simulink model "ROBOT"  (R2017a)
settings: Solver=VariableStepAuto  StartTime=0.0  StopTime=inf  MaxStep=0.05  RelTol=1e-3
model workspace: external: MATLAB File C:\Users\Robotic\Desktop\robot_solid\robot matlab\新建文件夹\ROBOT_DataFile.m (data not in the file)
values from neighbouring files (symbols this model uses):
  m = linspace(SD_4(1,30),SD_4(1,2),10)    [Gait_walking_go.m]
  X = A\B    [orbit_function.m]
  Y = 25*sin(2*pi/T*t)    [Gait_walkin.m]    (also in Gait_walking.m = 5*sin(2*pi/T*t); Gait_walking_go.m = 40*sin(2*pi/T*t))
undefined symbols (not defined in the file or in its folder): smiData, Z
libraries: sm_lib x579, nesl_utility x24, sldrtlib x1
(part 1 of 11)
settings Model: Creator=Robotic  LastModifiedBy=Administrator

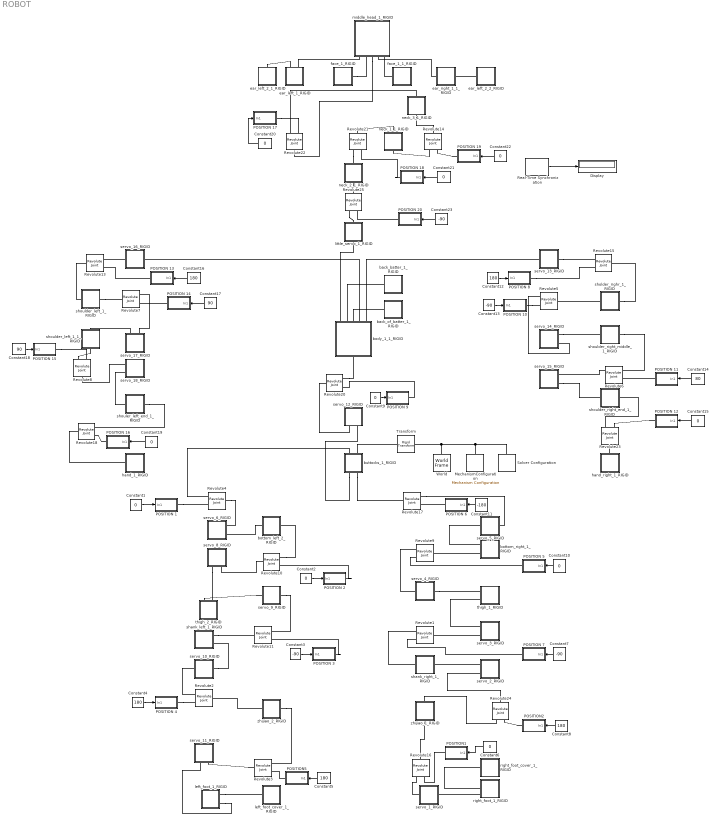
== system ROBOT ==
  Constant{1..2,6,9..10,15,19..22} (10 alike) : Constant  Value=0
  Constant11 : Constant  Value=-180
  Constant{4..5,8,12,16} (5 alike) : Constant  Value=180
  Constant{3,7,13,23} (4 alike) : Constant  Value=-90
  Constant14 : Constant  Value=80
  Constant17 : Constant  Value=90
  Constant18 : Constant  Value=90
  Display : Display
  MechanismConfiguration : sm_lib/Utilities/Mechanism Configuration  UniformGravity=Constant  GravityVector=[0 -9.80665 0]  GravityUnits=m/s^2  LinearizationDelta=0.001
  POSITION 1 : Subsystem
  POSITION 10 : Subsystem
  POSITION 11 : Subsystem
  POSITION 12 : Subsystem
  POSITION 13 : Subsystem
  POSITION 14 : Subsystem
  POSITION 15 : Subsystem
  POSITION 16 : Subsystem
  POSITION 17 : Subsystem
  POSITION 18 : Subsystem
  POSITION 19 : Subsystem
  POSITION 2 : Subsystem
  POSITION 20 : Subsystem
  POSITION 3 : Subsystem
  POSITION 4 : Subsystem
  POSITION 5 : Subsystem
  POSITION 6 : Subsystem
  POSITION 7 : Subsystem
  POSITION 8 : Subsystem
  POSITION 9 : Subsystem
  POSITION1 : Subsystem
  POSITION2 : Subsystem
  POSITION5 : Subsystem
  Real-Time Synchronization : sldrtlib/Real-Time Synchronization  SampleTime=0.1  MaxMissedTicks=100  ShowMissedTicks=on  YieldWhenWaiting=off
  Revolute{1..3,5,7..9,11,13..18,21..25} (19 alike) : sm_lib/Joints/Revolute Joint  SenseConstraintForce=off  SenseConstraintForceX=off  SenseConstraintForceY=off  SenseConstraintForceZ=off  SenseConstraintTorque=off  SenseConstraintTorqueX=off  SenseConstraintTorqueY=off  SenseConstraintTorqueZ=off  SenseTotalForce=off  SenseTotalForceX=off  SenseTotalForceY=off  SenseTotalForceZ=off  SenseTotalTorque=off  SenseTotalTorqueX=off  SenseTotalTorqueY=off  SenseTotalTorqueZ=off  CompositeWrenchDir=FollowerOnBase  CompositeWrenchFrame=BaseFrame  EquilibriumPosition=0  EquilibriumPositionUnits=rad  SpringStiffness=0  SpringStiffnessUnits=N*m/rad  DampingCoefficient=0  DampingCoefficientUnits=N*m/(rad/s)  TorqueActuationMode=ComputedTorque  MotionActuationMode=InputMotion  SensePosition=off  SenseVelocity=off  SenseAcceleration=off  SenseTorqueForce=off  PositionTargetSpecify=off  PositionTargetPriority=Low  PositionTargetValue=smiData.RevoluteJoint(2).Rz.Pos  PositionTargetValueUnits=deg  VelocityTargetSpecify=off  VelocityTargetPriority=High  VelocityTargetValue=0  VelocityTargetValueUnits=deg/s
  Revolute10 : sm_lib/Joints/Revolute Joint  SenseConstraintForce=off  SenseConstraintForceX=off  SenseConstraintForceY=off  SenseConstraintForceZ=off  SenseConstraintTorque=off  SenseConstraintTorqueX=off  SenseConstraintTorqueY=off  SenseConstraintTorqueZ=off  SenseTotalForce=off  SenseTotalForceX=off  SenseTotalForceY=off  SenseTotalForceZ=off  SenseTotalTorque=off  SenseTotalTorqueX=off  SenseTotalTorqueY=off  SenseTotalTorqueZ=off  CompositeWrenchDir=FollowerOnBase  CompositeWrenchFrame=BaseFrame  EquilibriumPosition=0  EquilibriumPositionUnits=rad  SpringStiffness=0  SpringStiffnessUnits=N*m/rad  DampingCoefficient=0  DampingCoefficientUnits=N*m/(rad/s)  TorqueActuationMode=ComputedTorque  MotionActuationMode=InputMotion  SensePosition=off  SenseVelocity=off  SenseAcceleration=off  SenseTorqueForce=off  PositionTargetSpecify=on  PositionTargetPriority=Low  PositionTargetValue=smiData.RevoluteJoint(2).Rz.Pos  PositionTargetValueUnits=deg  VelocityTargetSpecify=off  VelocityTargetPriority=High  VelocityTargetValue=0  VelocityTargetValueUnits=deg/s
  Revolute20 : sm_lib/Joints/Revolute Joint  SenseConstraintForce=off  SenseConstraintForceX=off  SenseConstraintForceY=off  SenseConstraintForceZ=off  SenseConstraintTorque=off  SenseConstraintTorqueX=off  SenseConstraintTorqueY=off  SenseConstraintTorqueZ=off  SenseTotalForce=off  SenseTotalForceX=off  SenseTotalForceY=off  SenseTotalForceZ=off  SenseTotalTorque=off  SenseTotalTorqueX=off  SenseTotalTorqueY=off  SenseTotalTorqueZ=off  CompositeWrenchDir=FollowerOnBase  CompositeWrenchFrame=BaseFrame  EquilibriumPosition=0  EquilibriumPositionUnits=rad  SpringStiffness=0  SpringStiffnessUnits=N*m/rad  DampingCoefficient=0  DampingCoefficientUnits=N*m/(rad/s)  TorqueActuationMode=ComputedTorque  MotionActuationMode=InputMotion  SensePosition=off  SenseVelocity=off  SenseAcceleration=off  SenseTorqueForce=off  PositionTargetSpecify=on  PositionTargetPriority=Low  PositionTargetValue=smiData.RevoluteJoint(2).Rz.Pos  PositionTargetValueUnits=deg  VelocityTargetSpecify=off  VelocityTargetPriority=High  VelocityTargetValue=0  VelocityTargetValueUnits=deg/s
  Revolute4 : sm_lib/Joints/Revolute Joint  SenseConstraintForce=off  SenseConstraintForceX=off  SenseConstraintForceY=off  SenseConstraintForceZ=off  SenseConstraintTorque=off  SenseConstraintTorqueX=off  SenseConstraintTorqueY=off  SenseConstraintTorqueZ=off  SenseTotalForce=off  SenseTotalForceX=off  SenseTotalForceY=off  SenseTotalForceZ=off  SenseTotalTorque=off  SenseTotalTorqueX=off  SenseTotalTorqueY=off  SenseTotalTorqueZ=off  CompositeWrenchDir=FollowerOnBase  CompositeWrenchFrame=BaseFrame  EquilibriumPosition=0  EquilibriumPositionUnits=rad  SpringStiffness=0  SpringStiffnessUnits=N*m/rad  DampingCoefficient=0  DampingCoefficientUnits=N*m/(rad/s)  TorqueActuationMode=ComputedTorque  MotionActuationMode=InputMotion  SensePosition=off  SenseVelocity=off  SenseAcceleration=off  SenseTorqueForce=off  PositionTargetSpecify=on  PositionTargetPriority=Low  PositionTargetValue=smiData.RevoluteJoint(2).Rz.Pos  PositionTargetValueUnits=deg  VelocityTargetSpecify=off  VelocityTargetPriority=High  VelocityTargetValue=0  VelocityTargetValueUnits=deg/s
  Revolute6 : sm_lib/Joints/Revolute Joint  SenseConstraintForce=off  SenseConstraintForceX=off  SenseConstraintForceY=off  SenseConstraintForceZ=off  SenseConstraintTorque=off  SenseConstraintTorqueX=off  SenseConstraintTorqueY=off  SenseConstraintTorqueZ=off  SenseTotalForce=off  SenseTotalForceX=off  SenseTotalForceY=off  SenseTotalForceZ=off  SenseTotalTorque=off  SenseTotalTorqueX=off  SenseTotalTorqueY=off  SenseTotalTorqueZ=off  CompositeWrenchDir=FollowerOnBase  CompositeWrenchFrame=BaseFrame  EquilibriumPosition=0  EquilibriumPositionUnits=rad  SpringStiffness=0  SpringStiffnessUnits=N*m/rad  DampingCoefficient=0  DampingCoefficientUnits=N*m/(rad/s)  TorqueActuationMode=ComputedTorque  MotionActuationMode=InputMotion  SensePosition=on  SenseVelocity=off  SenseAcceleration=off  SenseTorqueForce=off  PositionTargetSpecify=off  PositionTargetPriority=Low  PositionTargetValue=smiData.RevoluteJoint(2).Rz.Pos  PositionTargetValueUnits=deg  VelocityTargetSpecify=off  VelocityTargetPriority=High  VelocityTargetValue=0  VelocityTargetValueUnits=deg/s
  Solver Configuration : nesl_utility/Solver Configuration  PhysicalDomain=network_engine_domain  SubClassName=solver  LeftPortType=input  RightPortType=generic  Accelerate=off  Tones=[]  Harmonics=[]  SimulateNoise=off  Profile=off  UseLocalSampling=off  EnableSwitchedLinearOptims=on  FrequencyDomain=off  UseCCode=off  RelTol=0.001  AbsTol=1e-06  MinStep=1e-09  ToWorkspace=off  RevertToSquareIcSolve=off  NumHomotopyIterations=100  PhasorMode=off  PhasorModeNumHarmonics=1  OverrideAbsTol=off  DoDC=off  ResidualTolerance=1e-09  UseLocalSolver=off  LocalSolverChoice=NE_BACKWARD_EULER_ADVANCER  LocalSolverSampleTime=0.001  DoFixedCost=off  MaxNonlinIter=3  MaxModeIter=2  LinearAlgebra=Sparse  DelaysMemoryBudget=1024  AutomaticFiltering=on  FilteringTimeConstant=0.001
  Transform : sm_lib/Frames and Transforms/Rigid Transform  TranslationMethod=Cartesian  TranslationStandardOffset=0  TranslationLengthUnit=mm  TranslationStandardAxis=+Z  TranslationCartesianOffset=smiData.RigidTransform(235).translation  TranslationROffset=0  TranslationROffsetUnits=m  TranslationZOffset=0  TranslationZOffsetUnits=m  TranslationThetaOffset=0  TranslationThetaOffsetUnits=deg  RotationMethod=ArbitraryAxis  RotationAngleUnits=rad  RotationStandardAxis=+Z  RotationAngle=smiData.RigidTransform(235).angle  RotationArbitraryAxis=smiData.RigidTransform(235).axis  FollAlignAxisA=+X  BaseAlignAxisA=+Y  FollAlignAxisB=+Y  BaseAlignAxisB=+Z  RotationSequenceAxes=FollowerAxes  RotationSequence=XYX  RotationSequenceAngles=[0 0 0]  RotationSequenceAnglesUnits=deg  RotationMatrix=[1 0 0; 0 1 0; 0 0 1]
  World : sm_lib/Frames and Transforms/World Frame
  back_batter_1_RIGID : Subsystem
  back_of_batter_1_RIGID : Subsystem
  body_1_1_RIGID : Subsystem
  bottom_left_2_RIGID : Subsystem
  bottom_right_1_RIGID : Subsystem
  buttocks_1_RIGID : Subsystem
  ear_left_1_RIGID : Subsystem
  ear_left_2_1_RIGID : Subsystem
  ear_left_2_2_RIGID : Subsystem
  ear_right_1_1_RIGID : Subsystem
  face_1_1_RIGID : Subsystem
  face_1_RIGID : Subsystem
  hand_1_RIGID : Subsystem
  hand_right_1_RIGID : Subsystem
  left_foot_1_RIGID : Subsystem
  left_foot_cover_1_RIGID : Subsystem
  little_servo_1_RIGID : Subsystem
  middle_head_1_RIGID : Subsystem
  neck_1_1_RIGID : Subsystem
  neck_2_1_RIGID : Subsystem
  neck_3_1_RIGID : Subsystem
  right_foot_1_RIGID : Subsystem
  right_foot_cover_1_RIGID : Subsystem
  servo_10_RIGID : Subsystem
  servo_11_RIGID : Subsystem
  servo_12_RIGID : Subsystem
  servo_13_RIGID : Subsystem
  servo_14_RIGID : Subsystem
  servo_15_RIGID : Subsystem
  servo_16_RIGID : Subsystem
  servo_17_RIGID : Subsystem
  servo_18_RIGID : Subsystem
  servo_1_RIGID : Subsystem
  servo_2_RIGID : Subsystem
  servo_3_RIGID : Subsystem
  servo_4_RIGID : Subsystem
  servo_5_RIGID : Subsystem
  servo_6_RIGID : Subsystem
  servo_8_RIGID : Subsystem
  servo_9_RIGID : Subsystem
  shank_left_1_RIGID : Subsystem
  shank_right_1_RIGID : Subsystem
  sholder_righr_1_RIGID : Subsystem
  shoulder_left_1_1_RIGID : Subsystem
  shoulder_left_1_RIGID : Subsystem
  shoulder_right_end_1_RIGID : Subsystem
  shoulder_right_middle_1_RIGID : Subsystem
  shouler_left_end_1_RIGID : Subsystem
  thigh_1_RIGID : Subsystem
  thigh_2_RIGID : Subsystem
  zhijiao_1_RIGID : Subsystem
  zhijiao_2_RIGID : Subsystem
  wires:
  Constant7/1 -> POSITION 7/1(In1)
  Constant9/1 -> POSITION 9/1(In1)
  Constant1/1 -> POSITION 1/1(In1)
  Constant2/1 -> POSITION 2/1(In1)
  Constant3/1 -> POSITION 3/1(In1)
  Constant4/1 -> POSITION 4/1(In1)
  Constant5/1 -> POSITION5/1(In1)
  Constant6/1 -> POSITION1/1(In1)
  Constant8/1 -> POSITION2/1(In1)
  Constant10/1 -> POSITION 5/1(In1)
  Constant11/1 -> POSITION 6/1(In1)
  Constant12/1 -> POSITION 8/1(In1)
  Constant13/1 -> POSITION 10/1(In1)
  Constant14/1 -> POSITION 11/1(In1)
  Constant15/1 -> POSITION 12/1(In1)
  Constant16/1 -> POSITION 13/1(In1)
  Constant17/1 -> POSITION 14/1(In1)
  Constant18/1 -> POSITION 15/1(In1)
  Constant19/1 -> POSITION 16/1(In1)
  Constant20/1 -> POSITION 17/1(In1)
  Constant21/1 -> POSITION 18/1(In1)
  Constant22/1 -> POSITION 19/1(In1)
  Constant23/1 -> POSITION 20/1(In1)
  Real-Time Synchronization/1 -> Display/1
  connections:
  left_foot_1_RIGID/LConn2 -- servo_11_RIGID/LConn1
  body_1_1_RIGID/LConn5 -- servo_13_RIGID/LConn1
  servo_13_RIGID/RConn1 -- Revolute15/LConn1
  sholder_righr_1_RIGID/LConn1 -- Revolute15/RConn1
  sholder_righr_1_RIGID/RConn1 -- Revolute5/RConn1
  Revolute5/LConn1 -- servo_14_RIGID/LConn2
  servo_15_RIGID/LConn2 -- shoulder_right_end_1_RIGID/LConn1
  body_1_1_RIGID/LConn4 -- servo_16_RIGID/LConn1
  zhijiao_1_RIGID/LConn1 -- Revolute16/RConn1
  servo_16_RIGID/RConn1 -- Revolute13/LConn1
  shoulder_left_1_RIGID/LConn1 -- Revolute13/RConn1
  shoulder_left_1_RIGID/RConn1 -- Revolute7/RConn1
  servo_17_RIGID/LConn2 -- Revolute7/LConn1
  servo_18_RIGID/LConn2 -- shouler_left_end_1_RIGID/LConn1
  back_of_batter_1_RIGID/LConn1 -- body_1_1_RIGID/LConn3
  right_foot_1_RIGID/LConn3 -- servo_1_RIGID/LConn1
  right_foot_1_RIGID/LConn2 -- right_foot_cover_1_RIGID/LConn1
  servo_2_RIGID/LConn1 -- shank_right_1_RIGID/LConn1
  servo_3_RIGID/LConn1 -- thigh_1_RIGID/LConn2
  zhijiao_1_RIGID/RConn1 -- Revolute24/LConn1
  shank_right_1_RIGID/RConn1 -- Revolute1/LConn1
  servo_3_RIGID/LConn2 -- Revolute1/RConn1
  servo_4_RIGID/LConn1 -- thigh_1_RIGID/LConn1
  bottom_left_2_RIGID/LConn1 -- servo_6_RIGID/LConn2
  Revolute10/LConn1 -- bottom_left_2_RIGID/RConn1
  Revolute10/RConn1 -- servo_8_RIGID/LConn2
  servo_8_RIGID/LConn1 -- thigh_2_RIGID/LConn2
  servo_9_RIGID/LConn1 -- thigh_2_RIGID/LConn1
  servo_9_RIGID/RConn1 -- Revolute11/LConn1
  shank_left_1_RIGID/LConn1 -- Revolute11/RConn1
  servo_2_RIGID/LConn2 -- Revolute24/RConn1
  back_batter_1_RIGID/LConn1 -- body_1_1_RIGID/LConn2
  shouler_left_end_1_RIGID/RConn1 -- Revolute18/LConn1
  hand_1_RIGID/LConn1 -- Revolute18/RConn1
  left_foot_1_RIGID/LConn1 -- left_foot_cover_1_RIGID/LConn1
  Revolute23/LConn1 -- shoulder_right_end_1_RIGID/RConn1
  hand_right_1_RIGID/LConn1 -- Revolute23/RConn1
  body_1_1_RIGID/LConn1 -- little_servo_1_RIGID/LConn1
  Revolute25/LConn1 -- little_servo_1_RIGID/RConn1
  Revolute25/RConn1 -- neck_2_1_RIGID/LConn1
  buttocks_1_RIGID/LConn1 -- servo_12_RIGID/LConn2
  Revolute17/LConn1 -- servo_5_RIGID/RConn1
  buttocks_1_RIGID/LConn2 -- Revolute17/RConn1
  Revolute4/RConn1 -- servo_6_RIGID/LConn1
  face_1_1_RIGID/LConn1 -- middle_head_1_RIGID/LConn5
  servo_4_RIGID/RConn1 -- Revolute9/LConn1
  bottom_right_1_RIGID/LConn2 -- Revolute9/RConn1
  bottom_right_1_RIGID/LConn1 -- servo_5_RIGID/LConn1
  servo_17_RIGID/LConn1 -- shoulder_left_1_1_RIGID/LConn1
  shoulder_left_1_1_RIGID/RConn1 -- Revolute8/LConn1
  zhijiao_2_RIGID/LConn1 -- Revolute2/RConn1
  servo_18_RIGID/LConn1 -- Revolute8/RConn1
  ear_right_1_1_RIGID/LConn1 -- middle_head_1_RIGID/LConn4
  face_1_RIGID/LConn1 -- middle_head_1_RIGID/LConn2
  ear_left_1_RIGID/LConn2 -- middle_head_1_RIGID/LConn1
  neck_3_1_RIGID/RConn1 -- Revolute22/LConn1
  middle_head_1_RIGID/LConn3 -- Revolute22/RConn1
  ear_left_1_RIGID/LConn1 -- ear_left_2_1_RIGID/LConn1
  ear_left_2_2_RIGID/LConn1 -- ear_right_1_1_RIGID/RConn1
  Revolute21/LConn1 -- neck_2_1_RIGID/RConn1
  zhijiao_2_RIGID/RConn1 -- Revolute3/LConn1
  neck_1_1_RIGID/LConn1 -- Revolute21/RConn1
  Revolute14/LConn1 -- neck_1_1_RIGID/RConn1
  neck_3_1_RIGID/LConn1 -- Revolute14/RConn1
  servo_14_RIGID/LConn1 -- shoulder_right_middle_1_RIGID/LConn1
  shoulder_right_middle_1_RIGID/RConn1 -- Revolute6/LConn1
  Revolute6/RConn1 -- servo_15_RIGID/LConn1
  Revolute3/RConn1 -- servo_11_RIGID/LConn2
  servo_10_RIGID/LConn1 -- shank_left_1_RIGID/LConn2
  MechanismConfiguration/RConn1 -- Solver Configuration/RConn1 -- World/RConn1 -- Transform/LConn1
  Transform/RConn1 -- buttocks_1_RIGID/RConn2
  Revolute20/LConn1 -- body_1_1_RIGID/RConn1
  Revolute20/RConn1 -- servo_12_RIGID/LConn1
  POSITION 9/RConn1 -- Revolute20/LConn2
  buttocks_1_RIGID/RConn1 -- Revolute4/LConn1
  POSITION 1/RConn1 -- Revolute4/LConn2
  POSITION 2/RConn1 -- Revolute10/LConn2
  POSITION 3/RConn1 -- Revolute11/LConn2
  POSITION 4/RConn1 -- Revolute2/LConn2
  Revolute2/LConn1 -- servo_10_RIGID/RConn1
  POSITION5/RConn1 -- Revolute3/LConn2
  servo_1_RIGID/RConn1 -- Revolute16/LConn1
  POSITION1/RConn1 -- Revolute16/LConn2
  POSITION2/RConn1 -- Revolute24/LConn2
  POSITION 7/RConn1 -- Revolute1/LConn2
  POSITION 5/RConn1 -- Revolute9/LConn2
  POSITION 6/RConn1 -- Revolute17/LConn2
  POSITION 8/RConn1 -- Revolute15/LConn2
  POSITION 10/RConn1 -- Revolute5/LConn2
  POSITION 11/RConn1 -- Revolute6/LConn2
  POSITION 12/RConn1 -- Revolute23/LConn2
  POSITION 13/RConn1 -- Revolute13/LConn2
  POSITION 14/RConn1 -- Revolute7/LConn2
  POSITION 15/RConn1 -- Revolute8/LConn2
  POSITION 16/RConn1 -- Revolute18/LConn2
  POSITION 17/RConn1 -- Revolute22/LConn2
  POSITION 18/RConn1 -- Revolute21/LConn2
  POSITION 19/RConn1 -- Revolute14/LConn2
  POSITION 20/RConn1 -- Revolute25/LConn2

== system ROBOT/POSITION 1 ==
  In1 : Inport
  Constant : Constant  Value=0
  Gain : Gain  Gain=pi/180
  Simulink-PS Converter : nesl_utility/Simulink-PS Converter  PhysicalDomain=network_engine_domain  SubClassName=ps_input  LeftPortType=input  RightPortType=output  PseudoPeriodic=off  Frequencies=[]  NoiseDistribution=none  NoiseParameters=[]  Unit=rad  AffineConversion=off  FilteringAndDerivatives=provide  SimscapeFilterOrder=1  InputFilterTimeConstant=0.001  UdotUserProvided=0
  Subtract : Sum
  Conn1 : PMIOPort  Port=1  Side=Right
  wires:
  Gain/1 -> Simulink-PS Converter/1
  Constant/1 -> Subtract/2
  In1/1 -> Subtract/1
  Subtract/1 -> Gain/1
  connections:
  Simulink-PS Converter/RConn1 -- Conn1/RConn1

== system ROBOT/POSITION 10 ==
  In1 : Inport
  Constant : Constant  Value=0
  Gain : Gain  Gain=pi/180
  Simulink-PS Converter : nesl_utility/Simulink-PS Converter  PhysicalDomain=network_engine_domain  SubClassName=ps_input  LeftPortType=input  RightPortType=output  PseudoPeriodic=off  Frequencies=[]  NoiseDistribution=none  NoiseParameters=[]  Unit=rad  AffineConversion=off  FilteringAndDerivatives=provide  SimscapeFilterOrder=1  InputFilterTimeConstant=0.001  UdotUserProvided=0
  Subtract : Sum
  Conn1 : PMIOPort  Port=1  Side=Right
  wires:
  Gain/1 -> Simulink-PS Converter/1
  Constant/1 -> Subtract/2
  In1/1 -> Subtract/1
  Subtract/1 -> Gain/1
  connections:
  Simulink-PS Converter/RConn1 -- Conn1/RConn1

== system ROBOT/POSITION 11 ==
  In1 : Inport
  Constant : Constant  Value=0
  Gain : Gain  Gain=pi/180
  Simulink-PS Converter : nesl_utility/Simulink-PS Converter  PhysicalDomain=network_engine_domain  SubClassName=ps_input  LeftPortType=input  RightPortType=output  PseudoPeriodic=off  Frequencies=[]  NoiseDistribution=none  NoiseParameters=[]  Unit=rad  AffineConversion=off  FilteringAndDerivatives=provide  SimscapeFilterOrder=1  InputFilterTimeConstant=0.001  UdotUserProvided=0
  Subtract : Sum
  Conn1 : PMIOPort  Port=1  Side=Right
  wires:
  Gain/1 -> Simulink-PS Converter/1
  Constant/1 -> Subtract/2
  In1/1 -> Subtract/1
  Subtract/1 -> Gain/1
  connections:
  Simulink-PS Converter/RConn1 -- Conn1/RConn1

== system ROBOT/POSITION 12 ==
  In1 : Inport
  Constant : Constant  Value=0
  Gain : Gain  Gain=pi/180
  Simulink-PS Converter : nesl_utility/Simulink-PS Converter  PhysicalDomain=network_engine_domain  SubClassName=ps_input  LeftPortType=input  RightPortType=output  PseudoPeriodic=off  Frequencies=[]  NoiseDistribution=none  NoiseParameters=[]  Unit=rad  AffineConversion=off  FilteringAndDerivatives=provide  SimscapeFilterOrder=1  InputFilterTimeConstant=0.001  UdotUserProvided=0
  Subtract : Sum
  Conn1 : PMIOPort  Port=1  Side=Right
  wires:
  Gain/1 -> Simulink-PS Converter/1
  Constant/1 -> Subtract/2
  In1/1 -> Subtract/1
  Subtract/1 -> Gain/1
  connections:
  Simulink-PS Converter/RConn1 -- Conn1/RConn1

== system ROBOT/POSITION 13 ==
  In1 : Inport
  Constant : Constant  Value=0
  Gain : Gain  Gain=pi/180
  Simulink-PS Converter : nesl_utility/Simulink-PS Converter  PhysicalDomain=network_engine_domain  SubClassName=ps_input  LeftPortType=input  RightPortType=output  PseudoPeriodic=off  Frequencies=[]  NoiseDistribution=none  NoiseParameters=[]  Unit=rad  AffineConversion=off  FilteringAndDerivatives=provide  SimscapeFilterOrder=1  InputFilterTimeConstant=0.001  UdotUserProvided=0
  Subtract : Sum
  Conn1 : PMIOPort  Port=1  Side=Right
  wires:
  Gain/1 -> Simulink-PS Converter/1
  Constant/1 -> Subtract/2
  In1/1 -> Subtract/1
  Subtract/1 -> Gain/1
  connections:
  Simulink-PS Converter/RConn1 -- Conn1/RConn1

== system ROBOT/POSITION 14 ==
  In1 : Inport
  Constant : Constant  Value=0
  Gain : Gain  Gain=pi/180
  Simulink-PS Converter : nesl_utility/Simulink-PS Converter  PhysicalDomain=network_engine_domain  SubClassName=ps_input  LeftPortType=input  RightPortType=output  PseudoPeriodic=off  Frequencies=[]  NoiseDistribution=none  NoiseParameters=[]  Unit=rad  AffineConversion=off  FilteringAndDerivatives=provide  SimscapeFilterOrder=1  InputFilterTimeConstant=0.001  UdotUserProvided=0
  Subtract : Sum
  Conn1 : PMIOPort  Port=1  Side=Right
  wires:
  Gain/1 -> Simulink-PS Converter/1
  Constant/1 -> Subtract/2
  In1/1 -> Subtract/1
  Subtract/1 -> Gain/1
  connections:
  Simulink-PS Converter/RConn1 -- Conn1/RConn1

== system ROBOT/POSITION 15 ==
  In1 : Inport
  Constant : Constant  Value=0
  Gain : Gain  Gain=pi/180
  Simulink-PS Converter : nesl_utility/Simulink-PS Converter  PhysicalDomain=network_engine_domain  SubClassName=ps_input  LeftPortType=input  RightPortType=output  PseudoPeriodic=off  Frequencies=[]  NoiseDistribution=none  NoiseParameters=[]  Unit=rad  AffineConversion=off  FilteringAndDerivatives=provide  SimscapeFilterOrder=1  InputFilterTimeConstant=0.001  UdotUserProvided=0
  Subtract : Sum
  Conn1 : PMIOPort  Port=1  Side=Right
  wires:
  Gain/1 -> Simulink-PS Converter/1
  Constant/1 -> Subtract/2
  In1/1 -> Subtract/1
  Subtract/1 -> Gain/1
  connections:
  Simulink-PS Converter/RConn1 -- Conn1/RConn1

== system ROBOT/POSITION 16 ==
  In1 : Inport
  Constant : Constant  Value=0
  Gain : Gain  Gain=pi/180
  Simulink-PS Converter : nesl_utility/Simulink-PS Converter  PhysicalDomain=network_engine_domain  SubClassName=ps_input  LeftPortType=input  RightPortType=output  PseudoPeriodic=off  Frequencies=[]  NoiseDistribution=none  NoiseParameters=[]  Unit=rad  AffineConversion=off  FilteringAndDerivatives=provide  SimscapeFilterOrder=1  InputFilterTimeConstant=0.001  UdotUserProvided=0
  Subtract : Sum
  Conn1 : PMIOPort  Port=1  Side=Right
  wires:
  Gain/1 -> Simulink-PS Converter/1
  Constant/1 -> Subtract/2
  In1/1 -> Subtract/1
  Subtract/1 -> Gain/1
  connections:
  Simulink-PS Converter/RConn1 -- Conn1/RConn1

== system ROBOT/POSITION 17 ==
  In1 : Inport
  Constant : Constant  Value=0
  Gain : Gain  Gain=pi/180
  Simulink-PS Converter : nesl_utility/Simulink-PS Converter  PhysicalDomain=network_engine_domain  SubClassName=ps_input  LeftPortType=input  RightPortType=output  PseudoPeriodic=off  Frequencies=[]  NoiseDistribution=none  NoiseParameters=[]  Unit=rad  AffineConversion=off  FilteringAndDerivatives=provide  SimscapeFilterOrder=1  InputFilterTimeConstant=0.001  UdotUserProvided=0
  Subtract : Sum
  Conn1 : PMIOPort  Port=1  Side=Right
  wires:
  Gain/1 -> Simulink-PS Converter/1
  Constant/1 -> Subtract/2
  In1/1 -> Subtract/1
  Subtract/1 -> Gain/1
  connections:
  Simulink-PS Converter/RConn1 -- Conn1/RConn1

== system ROBOT/POSITION 18 ==
  In1 : Inport
  Constant : Constant  Value=0
  Gain : Gain  Gain=pi/180
  Simulink-PS Converter : nesl_utility/Simulink-PS Converter  PhysicalDomain=network_engine_domain  SubClassName=ps_input  LeftPortType=input  RightPortType=output  PseudoPeriodic=off  Frequencies=[]  NoiseDistribution=none  NoiseParameters=[]  Unit=rad  AffineConversion=off  FilteringAndDerivatives=provide  SimscapeFilterOrder=1  InputFilterTimeConstant=0.001  UdotUserProvided=0
  Subtract : Sum
  Conn1 : PMIOPort  Port=1  Side=Right
  wires:
  Gain/1 -> Simulink-PS Converter/1
  Constant/1 -> Subtract/2
  In1/1 -> Subtract/1
  Subtract/1 -> Gain/1
  connections:
  Simulink-PS Converter/RConn1 -- Conn1/RConn1

== system ROBOT/POSITION 19 ==
  In1 : Inport
  Constant : Constant  Value=0
  Gain : Gain  Gain=pi/180
  Simulink-PS Converter : nesl_utility/Simulink-PS Converter  PhysicalDomain=network_engine_domain  SubClassName=ps_input  LeftPortType=input  RightPortType=output  PseudoPeriodic=off  Frequencies=[]  NoiseDistribution=none  NoiseParameters=[]  Unit=rad  AffineConversion=off  FilteringAndDerivatives=provide  SimscapeFilterOrder=1  InputFilterTimeConstant=0.001  UdotUserProvided=0
  Subtract : Sum
  Conn1 : PMIOPort  Port=1  Side=Right
  wires:
  Gain/1 -> Simulink-PS Converter/1
  Constant/1 -> Subtract/2
  In1/1 -> Subtract/1
  Subtract/1 -> Gain/1
  connections:
  Simulink-PS Converter/RConn1 -- Conn1/RConn1

== system ROBOT/POSITION 2 ==
  In1 : Inport
  Constant : Constant  Value=0
  Gain : Gain  Gain=pi/180
  Simulink-PS Converter : nesl_utility/Simulink-PS Converter  PhysicalDomain=network_engine_domain  SubClassName=ps_input  LeftPortType=input  RightPortType=output  PseudoPeriodic=off  Frequencies=[]  NoiseDistribution=none  NoiseParameters=[]  Unit=rad  AffineConversion=off  FilteringAndDerivatives=provide  SimscapeFilterOrder=1  InputFilterTimeConstant=0.001  UdotUserProvided=0
  Subtract : Sum
  Conn1 : PMIOPort  Port=1  Side=Right
  wires:
  Gain/1 -> Simulink-PS Converter/1
  Constant/1 -> Subtract/2
  In1/1 -> Subtract/1
  Subtract/1 -> Gain/1
  connections:
  Simulink-PS Converter/RConn1 -- Conn1/RConn1

== system ROBOT/POSITION 20 ==
  In1 : Inport
  Constant : Constant  Value=0
  Gain : Gain  Gain=pi/180
  Simulink-PS Converter : nesl_utility/Simulink-PS Converter  PhysicalDomain=network_engine_domain  SubClassName=ps_input  LeftPortType=input  RightPortType=output  PseudoPeriodic=off  Frequencies=[]  NoiseDistribution=none  NoiseParameters=[]  Unit=rad  AffineConversion=off  FilteringAndDerivatives=provide  SimscapeFilterOrder=1  InputFilterTimeConstant=0.001  UdotUserProvided=0
  Subtract : Sum
  Conn1 : PMIOPort  Port=1  Side=Right
  wires:
  Gain/1 -> Simulink-PS Converter/1
  Constant/1 -> Subtract/2
  In1/1 -> Subtract/1
  Subtract/1 -> Gain/1
  connections:
  Simulink-PS Converter/RConn1 -- Conn1/RConn1

== system ROBOT/POSITION 3 ==
  In1 : Inport
  Constant : Constant  Value=0
  Gain : Gain  Gain=pi/180
  Simulink-PS Converter : nesl_utility/Simulink-PS Converter  PhysicalDomain=network_engine_domain  SubClassName=ps_input  LeftPortType=input  RightPortType=output  PseudoPeriodic=off  Frequencies=[]  NoiseDistribution=none  NoiseParameters=[]  Unit=rad  AffineConversion=off  FilteringAndDerivatives=provide  SimscapeFilterOrder=1  InputFilterTimeConstant=0.001  UdotUserProvided=0
  Subtract : Sum
  Conn1 : PMIOPort  Port=1  Side=Right
  wires:
  Gain/1 -> Simulink-PS Converter/1
  Constant/1 -> Subtract/2
  In1/1 -> Subtract/1
  Subtract/1 -> Gain/1
  connections:
  Simulink-PS Converter/RConn1 -- Conn1/RConn1

== system ROBOT/POSITION 4 ==
  In1 : Inport
  Constant : Constant  Value=0
  Gain : Gain  Gain=pi/180
  Simulink-PS Converter : nesl_utility/Simulink-PS Converter  PhysicalDomain=network_engine_domain  SubClassName=ps_input  LeftPortType=input  RightPortType=output  PseudoPeriodic=off  Frequencies=[]  NoiseDistribution=none  NoiseParameters=[]  Unit=rad  AffineConversion=off  FilteringAndDerivatives=provide  SimscapeFilterOrder=1  InputFilterTimeConstant=0.001  UdotUserProvided=0
  Subtract : Sum
  Conn1 : PMIOPort  Port=1  Side=Right
  wires:
  Gain/1 -> Simulink-PS Converter/1
  Constant/1 -> Subtract/2
  In1/1 -> Subtract/1
  Subtract/1 -> Gain/1
  connections:
  Simulink-PS Converter/RConn1 -- Conn1/RConn1

== system ROBOT/POSITION 5 ==
  In1 : Inport
  Constant : Constant  Value=0
  Gain : Gain  Gain=pi/180
  Simulink-PS Converter : nesl_utility/Simulink-PS Converter  PhysicalDomain=network_engine_domain  SubClassName=ps_input  LeftPortType=input  RightPortType=output  PseudoPeriodic=off  Frequencies=[]  NoiseDistribution=none  NoiseParameters=[]  Unit=rad  AffineConversion=off  FilteringAndDerivatives=provide  SimscapeFilterOrder=1  InputFilterTimeConstant=0.001  UdotUserProvided=0
  Subtract : Sum
  Conn1 : PMIOPort  Port=1  Side=Right
  wires:
  Gain/1 -> Simulink-PS Converter/1
  Constant/1 -> Subtract/2
  In1/1 -> Subtract/1
  Subtract/1 -> Gain/1
  connections:
  Simulink-PS Converter/RConn1 -- Conn1/RConn1

== system ROBOT/POSITION 6 ==
  In1 : Inport
  Constant : Constant  Value=0
  Gain : Gain  Gain=pi/180
  Simulink-PS Converter : nesl_utility/Simulink-PS Converter  PhysicalDomain=network_engine_domain  SubClassName=ps_input  LeftPortType=input  RightPortType=output  PseudoPeriodic=off  Frequencies=[]  NoiseDistribution=none  NoiseParameters=[]  Unit=rad  AffineConversion=off  FilteringAndDerivatives=provide  SimscapeFilterOrder=1  InputFilterTimeConstant=0.001  UdotUserProvided=0
  Subtract : Sum
  Conn1 : PMIOPort  Port=1  Side=Right
  wires:
  Gain/1 -> Simulink-PS Converter/1
  Constant/1 -> Subtract/2
  In1/1 -> Subtract/1
  Subtract/1 -> Gain/1
  connections:
  Simulink-PS Converter/RConn1 -- Conn1/RConn1

== system ROBOT/POSITION 7 ==
  In1 : Inport
  Constant : Constant  Value=0
  Gain : Gain  Gain=pi/180
  Simulink-PS Converter : nesl_utility/Simulink-PS Converter  PhysicalDomain=network_engine_domain  SubClassName=ps_input  LeftPortType=input  RightPortType=output  PseudoPeriodic=off  Frequencies=[]  NoiseDistribution=none  NoiseParameters=[]  Unit=rad  AffineConversion=off  FilteringAndDerivatives=provide  SimscapeFilterOrder=1  InputFilterTimeConstant=0.001  UdotUserProvided=0
  Subtract : Sum
  Conn1 : PMIOPort  Port=1  Side=Right
  wires:
  Gain/1 -> Simulink-PS Converter/1
  Constant/1 -> Subtract/2
  In1/1 -> Subtract/1
  Subtract/1 -> Gain/1
  connections:
  Simulink-PS Converter/RConn1 -- Conn1/RConn1

== system ROBOT/POSITION 8 ==
  In1 : Inport
  Constant : Constant  Value=0
  Gain : Gain  Gain=pi/180
  Simulink-PS Converter : nesl_utility/Simulink-PS Converter  PhysicalDomain=network_engine_domain  SubClassName=ps_input  LeftPortType=input  RightPortType=output  PseudoPeriodic=off  Frequencies=[]  NoiseDistribution=none  NoiseParameters=[]  Unit=rad  AffineConversion=off  FilteringAndDerivatives=provide  SimscapeFilterOrder=1  InputFilterTimeConstant=0.001  UdotUserProvided=0
  Subtract : Sum
  Conn1 : PMIOPort  Port=1  Side=Right
  wires:
  Gain/1 -> Simulink-PS Converter/1
  Constant/1 -> Subtract/2
  In1/1 -> Subtract/1
  Subtract/1 -> Gain/1
  connections:
  Simulink-PS Converter/RConn1 -- Conn1/RConn1

== system ROBOT/POSITION 9 ==
  In1 : Inport
  Constant : Constant  Value=0
  Gain : Gain  Gain=pi/180
  Simulink-PS Converter : nesl_utility/Simulink-PS Converter  PhysicalDomain=network_engine_domain  SubClassName=ps_input  LeftPortType=input  RightPortType=output  PseudoPeriodic=off  Frequencies=[]  NoiseDistribution=none  NoiseParameters=[]  Unit=rad  AffineConversion=off  FilteringAndDerivatives=provide  SimscapeFilterOrder=1  InputFilterTimeConstant=0.001  UdotUserProvided=0
  Subtract : Sum
  Conn1 : PMIOPort  Port=1  Side=Right
  wires:
  Gain/1 -> Simulink-PS Converter/1
  Constant/1 -> Subtract/2
  In1/1 -> Subtract/1
  Subtract/1 -> Gain/1
  connections:
  Simulink-PS Converter/RConn1 -- Conn1/RConn1

== system ROBOT/POSITION1 ==
  In1 : Inport
  Constant : Constant  Value=0
  Gain : Gain  Gain=pi/180
  Simulink-PS Converter : nesl_utility/Simulink-PS Converter  PhysicalDomain=network_engine_domain  SubClassName=ps_input  LeftPortType=input  RightPortType=output  PseudoPeriodic=off  Frequencies=[]  NoiseDistribution=none  NoiseParameters=[]  Unit=rad  AffineConversion=off  FilteringAndDerivatives=provide  SimscapeFilterOrder=1  InputFilterTimeConstant=0.001  UdotUserProvided=0
  Subtract : Sum
  Conn1 : PMIOPort  Port=1  Side=Right
  wires:
  Gain/1 -> Simulink-PS Converter/1
  Constant/1 -> Subtract/2
  In1/1 -> Subtract/1
  Subtract/1 -> Gain/1
  connections:
  Simulink-PS Converter/RConn1 -- Conn1/RConn1

== system ROBOT/POSITION2 ==
  In1 : Inport
  Constant : Constant  Value=0
  Gain : Gain  Gain=pi/180
  Simulink-PS Converter : nesl_utility/Simulink-PS Converter  PhysicalDomain=network_engine_domain  SubClassName=ps_input  LeftPortType=input  RightPortType=output  PseudoPeriodic=off  Frequencies=[]  NoiseDistribution=none  NoiseParameters=[]  Unit=rad  AffineConversion=off  FilteringAndDerivatives=provide  SimscapeFilterOrder=1  InputFilterTimeConstant=0.001  UdotUserProvided=0
  Subtract : Sum
  Conn1 : PMIOPort  Port=1  Side=Right
  wires:
  Gain/1 -> Simulink-PS Converter/1
  Constant/1 -> Subtract/2
  In1/1 -> Subtract/1
  Subtract/1 -> Gain/1
  connections:
  Simulink-PS Converter/RConn1 -- Conn1/RConn1

== system ROBOT/POSITION5 ==
  In1 : Inport
  Constant : Constant  Value=0
  Gain : Gain  Gain=pi/180
  Simulink-PS Converter : nesl_utility/Simulink-PS Converter  PhysicalDomain=network_engine_domain  SubClassName=ps_input  LeftPortType=input  RightPortType=output  PseudoPeriodic=off  Frequencies=[]  NoiseDistribution=none  NoiseParameters=[]  Unit=rad  AffineConversion=off  FilteringAndDerivatives=provide  SimscapeFilterOrder=1  InputFilterTimeConstant=0.001  UdotUserProvided=0
  Subtract : Sum
  Conn1 : PMIOPort  Port=1  Side=Right
  wires:
  Gain/1 -> Simulink-PS Converter/1
  Constant/1 -> Subtract/2
  In1/1 -> Subtract/1
  Subtract/1 -> Gain/1
  connections:
  Simulink-PS Converter/RConn1 -- Conn1/RConn1

== system ROBOT/back_batter_1_RIGID ==
  ReferenceFrame : sm_lib/Frames and Transforms/Reference Frame
  Solid : sm_lib/Body Elements/Solid  InertiaType=Custom  Mass=smiData.Solid(82).mass  MassUnits=kg  CenterOfMass=smiData.Solid(82).CoM  CenterOfMassUnits=mm  MomentsOfInertia=smiData.Solid(82).MoI  MomentsOfInertiaUnits=kg*mm^2  ProductsOfInertia=smiData.Solid(82).PoI  ProductsOfInertiaUnits=kg*mm^2  DensityBased=on  Density=1000  DensityUnits=kg/m^3  DoExposeReferenceFrame=on  SerializedFrames=<Frames/>  GraphicType=FromGeometry  MarkerShape=Sphere  MarkerSize=10  GraphicVisPropType=SimpleVisualProperties  GraphicDiffuseColor=smiData.Solid(82).color  GraphicSpecularColor=[0.5 0.5 0.5 1.0]  GraphicAmbientColor=[0.15 0.15 0.15 1.0]  GraphicEmissiveColor=[0.0 0.0 0.0 1.0]  GraphicShininess=75  GraphicOpacity=smiData.Solid(82).opacity  GeometryShape=FromFile  RectangleSize=[1 1]  RectangleSizeUnits=m  BrickDimensions=[1 1 1]  BrickDimensionUnits=m  CylinderRadius=1  CylinderRadiusUnits=m  CylinderLength=1  CylinderLengthUnits=m  SphereRadius=1  SphereRadiusUnits=m  EllipsoidRadii=[1 1 1]  EllipsoidRadiiUnits=m  ExtrusionCrossSection=[1 1; -1 1; -1 -1; 1 -1]  ExtrusionCrossSectionUnits=m  ExtrusionLength=1  ExtrusionLengthUnits=m  PolygonNumSides=3  PolygonOuterRadius=1  PolygonOuterRadiusUnits=m  ExtGeomFileType=STEP  ExtGeomFileName=back batter_Default_sldprt.STEP  ExtGeomFileUnits=m  RevolutionCrossSection=[1 1; 1 -1; 2 -1; 2 1]  RevolutionCrossSectionUnits=m  RevolutionExtent=Full  RevolutionAngle=180  RevolutionAngleUnits=deg
  Transform : sm_lib/Frames and Transforms/Rigid Transform  TranslationMethod=Cartesian  TranslationStandardOffset=0  TranslationLengthUnit=mm  TranslationStandardAxis=+Z  TranslationCartesianOffset=smiData.RigidTransform(56).translation  TranslationROffset=0  TranslationROffsetUnits=m  TranslationZOffset=0  TranslationZOffsetUnits=m  TranslationThetaOffset=0  TranslationThetaOffsetUnits=deg  RotationMethod=ArbitraryAxis  RotationAngleUnits=rad  RotationStandardAxis=+Z  RotationAngle=smiData.RigidTransform(56).angle  RotationArbitraryAxis=smiData.RigidTransform(56).axis  FollAlignAxisA=+X  BaseAlignAxisA=+Y  FollAlignAxisB=+Y  BaseAlignAxisB=+Z  RotationSequenceAxes=FollowerAxes  RotationSequence=XYX  RotationSequenceAngles=[0 0 0]  RotationSequenceAnglesUnits=deg  RotationMatrix=[1 0 0; 0 1 0; 0 0 1]
  F : PMIOPort  Port=1  Side=Left
  connections:
  Solid/RConn1 -- ReferenceFrame/RConn1 -- Transform/LConn1
  Transform/RConn1 -- F/RConn1

== system ROBOT/back_of_batter_1_RIGID ==
  ReferenceFrame : sm_lib/Frames and Transforms/Reference Frame
  Solid : sm_lib/Body Elements/Solid  InertiaType=Custom  Mass=smiData.Solid(89).mass  MassUnits=kg  CenterOfMass=smiData.Solid(89).CoM  CenterOfMassUnits=mm  MomentsOfInertia=smiData.Solid(89).MoI  MomentsOfInertiaUnits=kg*mm^2  ProductsOfInertia=smiData.Solid(89).PoI  ProductsOfInertiaUnits=kg*mm^2  DensityBased=on  Density=1000  DensityUnits=kg/m^3  DoExposeReferenceFrame=on  SerializedFrames=<Frames/>  GraphicType=FromGeometry  MarkerShape=Sphere  MarkerSize=10  GraphicVisPropType=SimpleVisualProperties  GraphicDiffuseColor=smiData.Solid(89).color  GraphicSpecularColor=[0.5 0.5 0.5 1.0]  GraphicAmbientColor=[0.15 0.15 0.15 1.0]  GraphicEmissiveColor=[0.0 0.0 0.0 1.0]  GraphicShininess=75  GraphicOpacity=smiData.Solid(89).opacity  GeometryShape=FromFile  RectangleSize=[1 1]  RectangleSizeUnits=m  BrickDimensions=[1 1 1]  BrickDimensionUnits=m  CylinderRadius=1  CylinderRadiusUnits=m  CylinderLength=1  CylinderLengthUnits=m  SphereRadius=1  SphereRadiusUnits=m  EllipsoidRadii=[1 1 1]  EllipsoidRadiiUnits=m  ExtrusionCrossSection=[1 1; -1 1; -1 -1; 1 -1]  ExtrusionCrossSectionUnits=m  ExtrusionLength=1  ExtrusionLengthUnits=m  PolygonNumSides=3  PolygonOuterRadius=1  PolygonOuterRadiusUnits=m  ExtGeomFileType=STEP  ExtGeomFileName=back of batter_Default_sldprt.STEP  ExtGeomFileUnits=m  RevolutionCrossSection=[1 1; 1 -1; 2 -1; 2 1]  RevolutionCrossSectionUnits=m  RevolutionExtent=Full  RevolutionAngle=180  RevolutionAngleUnits=deg
  Transform : sm_lib/Frames and Transforms/Rigid Transform  TranslationMethod=Cartesian  TranslationStandardOffset=0  TranslationLengthUnit=mm  TranslationStandardAxis=+Z  TranslationCartesianOffset=smiData.RigidTransform(32).translation  TranslationROffset=0  TranslationROffsetUnits=m  TranslationZOffset=0  TranslationZOffsetUnits=m  TranslationThetaOffset=0  TranslationThetaOffsetUnits=deg  RotationMethod=ArbitraryAxis  RotationAngleUnits=rad  RotationStandardAxis=+Z  RotationAngle=smiData.RigidTransform(32).angle  RotationArbitraryAxis=smiData.RigidTransform(32).axis  FollAlignAxisA=+X  BaseAlignAxisA=+Y  FollAlignAxisB=+Y  BaseAlignAxisB=+Z  RotationSequenceAxes=FollowerAxes  RotationSequence=XYX  RotationSequenceAngles=[0 0 0]  RotationSequenceAnglesUnits=deg  RotationMatrix=[1 0 0; 0 1 0; 0 0 1]
  F : PMIOPort  Port=1  Side=Left
  connections:
  Solid/RConn1 -- ReferenceFrame/RConn1 -- Transform/LConn1
  Transform/RConn1 -- F/RConn1
